simulink model "Total_Pjt"  (R2023b)
settings: Solver=FixedStepAuto  StartTime=0.0  StopTime=10.0  RelTol=1e-3
values from neighbouring files (symbols this model uses):
  Ts = 0.01    [para.m]
settings Model: Creator=User  LastModifiedBy=User
settings OptimizationCC: DefaultParameterBehavior=Inlined  EnhancedBackFolding=on  PassReuseOutputArgsAs=Individual arguments  ZeroExternalMemoryAtStartup=off  ZeroInternalMemoryAtStartup=off  OptimizeBlockOrder=speed  DifferentSizesBufferReuse=on  OptimizationCustomize=off  EfficientTunableParamExpr=on
settings DebuggingCC: ParameterTunabilityLossMsg=error
settings SFSimCC: MATLABDynamicMemAlloc=off
settings RTWCC: Description=Embedded Coder  SystemTargetFile=ert.tlc  GenCodeOnly=on  TemplateMakefile=ert_default_tmf
settings CodeAppCC: ForceParamTrailComments=on  IgnoreCustomStorageClasses=off  OperatorAnnotations=on  SimulinkDataObjDesc=on  SFDataObjDesc=on  InsertBlockDesc=on
settings ERTTargetCC: TargetLangStandard=C99 (ISO)  GenerateSampleERTMain=on  InlinedParameterPlacement=NonHierarchical  ERTCustomFileTemplate=example_file_process.tlc

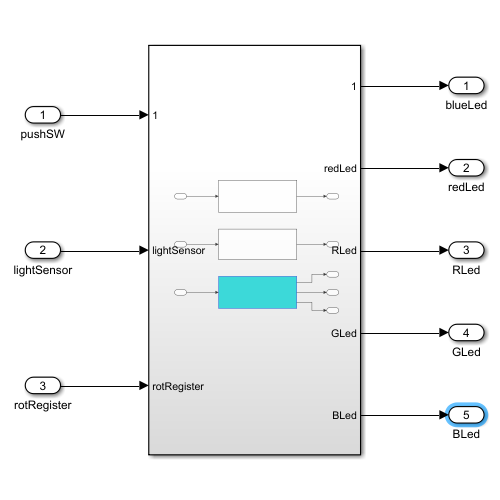
[thumbnail: Simulink's stored preview of the top-level diagram]
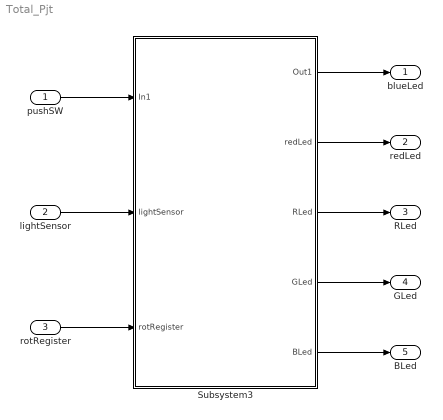
== system Total_Pjt ==
  pushSW : Inport  OutDataTypeStr=boolean
  lightSensor : Inport  Port=2
  rotRegister : Inport  Port=3
  Subsystem3 : Subsystem
  blueLed : Outport  OutDataTypeStr=uint16
  redLed : Outport  Port=2
  RLed : Outport  Port=3
  GLed : Outport  Port=4
  BLed : Outport  Port=5
  wires:
  pushSW/1 -> Subsystem3/1(In1)
  lightSensor/1 -> Subsystem3/2(lightSensor)
  rotRegister/1 -> Subsystem3/3(rotRegister)
  Subsystem3/1(Out1) -> blueLed/1
  Subsystem3/2(redLed) -> redLed/1
  Subsystem3/3(RLed) -> RLed/1
  Subsystem3/4(GLed) -> GLed/1
  Subsystem3/5(BLed) -> BLed/1

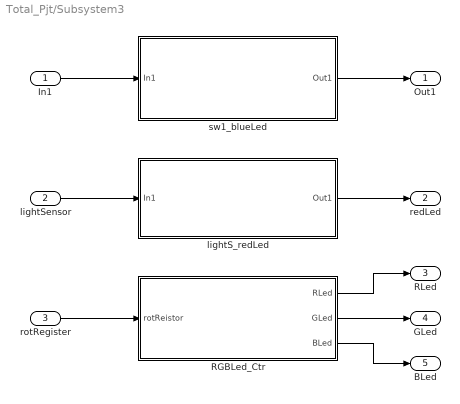
== system Total_Pjt/Subsystem3 ==
  In1 : Inport
  lightSensor : Inport  Port=2
  rotRegister : Inport  Port=3
  RGBLed_Ctr : Subsystem
  lightS_redLed : Subsystem
  sw1_blueLed : Subsystem
  Out1 : Outport
  redLed : Outport  Port=2
  RLed : Outport  Port=3
  GLed : Outport  Port=4
  BLed : Outport  Port=5
  wires:
  lightSensor/1 -> lightS_redLed/1(In1)
  In1/1 -> sw1_blueLed/1(In1)
  lightS_redLed/1(Out1) -> redLed/1
  sw1_blueLed/1(Out1) -> Out1/1
  rotRegister/1 -> RGBLed_Ctr/1(rotReistor)
  RGBLed_Ctr/1(RLed) -> RLed/1
  RGBLed_Ctr/2(GLed) -> GLed/1
  RGBLed_Ctr/3(BLed) -> BLed/1

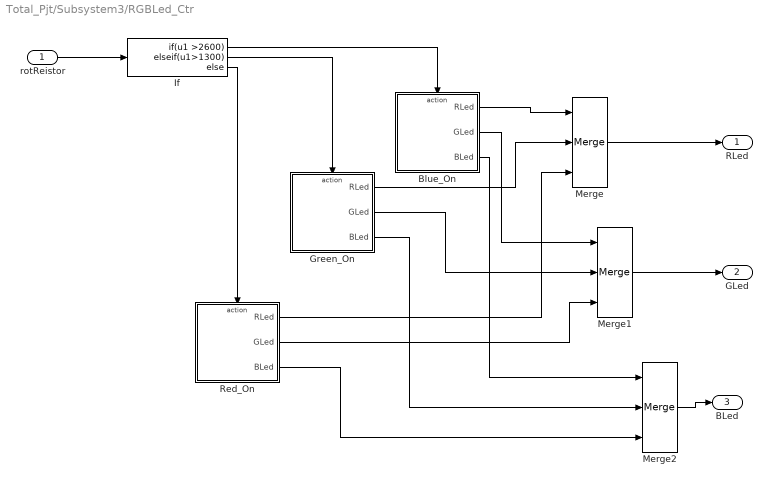
== system Total_Pjt/Subsystem3/RGBLed_Ctr ==
  rotReistor : Inport
  Blue_On : Subsystem  TreatAsAtomicUnit=on
  Green_On : Subsystem  TreatAsAtomicUnit=on
  If : If  IfExpression=u1 >2600  ElseIfExpressions=u1>1300
  Merge : Merge  Inputs=3
  Merge1 : Merge  Inputs=3
  Merge2 : Merge  Inputs=3
  Red_On : Subsystem  TreatAsAtomicUnit=on
  RLed : Outport
  GLed : Outport  Port=2
  BLed : Outport  Port=3
  wires:
  If/1 -> Blue_On/Action
  rotReistor/1 -> If/1
  If/2 -> Green_On/Action
  If/3 -> Red_On/Action
  Blue_On/1(RLed) -> Merge/1
  Green_On/1(RLed) -> Merge/2
  Blue_On/2(GLed) -> Merge1/1
  Green_On/2(GLed) -> Merge1/2
  Blue_On/3(BLed) -> Merge2/1
  Green_On/3(BLed) -> Merge2/2
  Red_On/3(BLed) -> Merge2/3
  Red_On/1(RLed) -> Merge/3
  Merge/1 -> RLed/1
  Red_On/2(GLed) -> Merge1/3
  Merge1/1 -> GLed/1
  Merge2/1 -> BLed/1

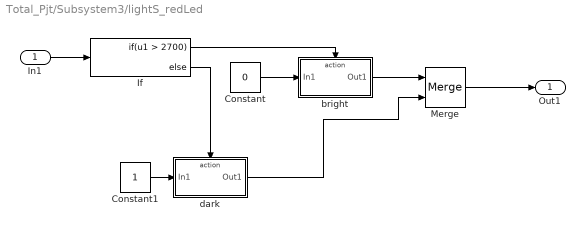
== system Total_Pjt/Subsystem3/lightS_redLed ==
  In1 : Inport
  Constant : Constant  Value=0
  Constant1 : Constant
  If : If  IfExpression=u1 > 2700
  Merge : Merge
  bright : Subsystem  TreatAsAtomicUnit=on
  dark : Subsystem  TreatAsAtomicUnit=on
  Out1 : Outport
  wires:
  dark/1(Out1) -> Merge/2
  bright/1(Out1) -> Merge/1
  Constant/1 -> bright/1(In1)
  If/1 -> bright/Action
  Constant1/1 -> dark/1(In1)
  In1/1 -> If/1
  Merge/1 -> Out1/1
  If/2 -> dark/Action

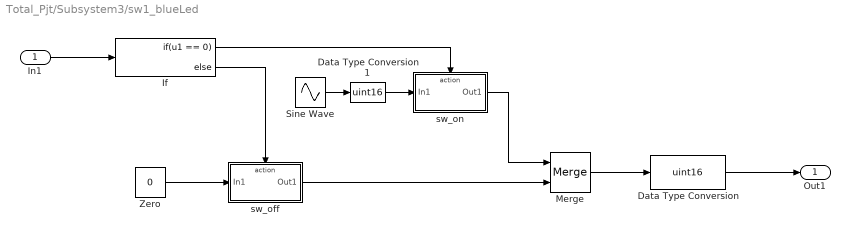
== system Total_Pjt/Subsystem3/sw1_blueLed ==
  In1 : Inport
  Data Type Conversion : DataTypeConversion  OutDataTypeStr=uint16  SaturateOnIntegerOverflow=off  RndMeth=Floor
  Data Type Conversion1 : DataTypeConversion  OutDataTypeStr=uint16  SaturateOnIntegerOverflow=off  RndMeth=Floor
  If : If  IfExpression=u1 == 0
  Merge : Merge
  Sine Wave : Sin  SineType=Sample based  Amplitude=25000  Bias=25000  Frequency=300  Samples=300  SampleTime=Ts
  Zero : Constant  Value=0  OutDataTypeStr=uint16
  sw_off : Subsystem  TreatAsAtomicUnit=on
  sw_on : Subsystem  TreatAsAtomicUnit=on
  Out1 : Outport
  wires:
  If/2 -> sw_off/Action
  Data Type Conversion1/1 -> sw_on/1(In1)
  Sine Wave/1 -> Data Type Conversion1/1
  Zero/1 -> sw_off/1(In1)
  If/1 -> sw_on/Action
  sw_off/1(Out1) -> Merge/2
  sw_on/1(Out1) -> Merge/1
  Merge/1 -> Data Type Conversion/1
  Data Type Conversion/1 -> Out1/1
  In1/1 -> If/1

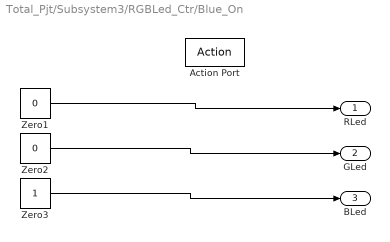
== system Total_Pjt/Subsystem3/RGBLed_Ctr/Blue_On ==
  Action Port : ActionPort  ActionPortLabel=if(u1 >2600)
  Zero1 : Constant  Value=0  OutDataTypeStr=boolean
  Zero2 : Constant  Value=0  OutDataTypeStr=boolean
  Zero3 : Constant  OutDataTypeStr=boolean
  RLed : Outport
  GLed : Outport  Port=2
  BLed : Outport  Port=3
  wires:
  Zero3/1 -> BLed/1
  Zero2/1 -> GLed/1
  Zero1/1 -> RLed/1

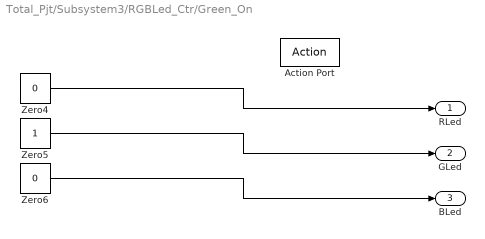
== system Total_Pjt/Subsystem3/RGBLed_Ctr/Green_On ==
  Action Port : ActionPort  ActionPortLabel=elseif(u1>1300)
  Zero4 : Constant  Value=0  OutDataTypeStr=boolean
  Zero5 : Constant  OutDataTypeStr=boolean
  Zero6 : Constant  Value=0  OutDataTypeStr=boolean
  RLed : Outport
  GLed : Outport  Port=2
  BLed : Outport  Port=3
  wires:
  Zero4/1 -> RLed/1
  Zero6/1 -> BLed/1
  Zero5/1 -> GLed/1

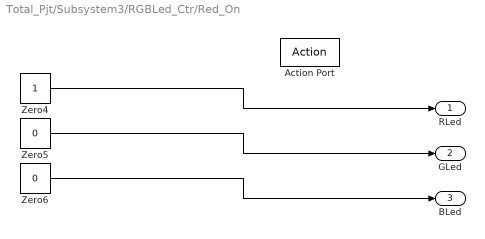
== system Total_Pjt/Subsystem3/RGBLed_Ctr/Red_On ==
  Action Port : ActionPort  ActionPortLabel=else
  Zero4 : Constant  OutDataTypeStr=boolean
  Zero5 : Constant  Value=0  OutDataTypeStr=boolean
  Zero6 : Constant  Value=0  OutDataTypeStr=boolean
  RLed : Outport
  GLed : Outport  Port=2
  BLed : Outport  Port=3
  wires:
  Zero5/1 -> GLed/1
  Zero6/1 -> BLed/1
  Zero4/1 -> RLed/1

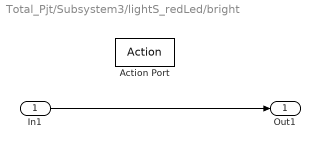
== system Total_Pjt/Subsystem3/lightS_redLed/bright ==
  In1 : Inport
  Action Port : ActionPort  ActionPortLabel=if(u1 > 2700)
  Out1 : Outport
  wires:
  In1/1 -> Out1/1

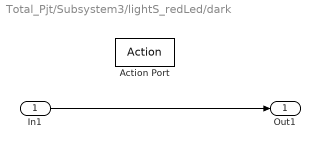
== system Total_Pjt/Subsystem3/lightS_redLed/dark ==
  In1 : Inport
  Action Port : ActionPort  ActionPortLabel=else
  Out1 : Outport
  wires:
  In1/1 -> Out1/1

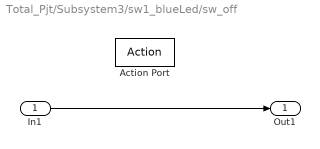
== system Total_Pjt/Subsystem3/sw1_blueLed/sw_off ==
  In1 : Inport  OutDataTypeStr=uint16
  Action Port : ActionPort  ActionPortLabel=else
  Out1 : Outport  OutDataTypeStr=uint16
  wires:
  In1/1 -> Out1/1

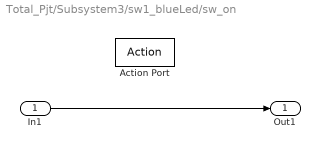
== system Total_Pjt/Subsystem3/sw1_blueLed/sw_on ==
  In1 : Inport  OutDataTypeStr=uint16
  Action Port : ActionPort  ActionPortLabel=if(u1 == 0)
  Out1 : Outport  OutDataTypeStr=uint16
  wires:
  In1/1 -> Out1/1
